simulink model "sampleModel1996"  (R2023a)
settings: Solver=VariableStepAuto  StartTime=0.0  StopTime=10.0  RelTol=1e-3
libraries: simulink x3, hdlsllib x2
settings Model: Creator=user1  LastModifiedBy=user1

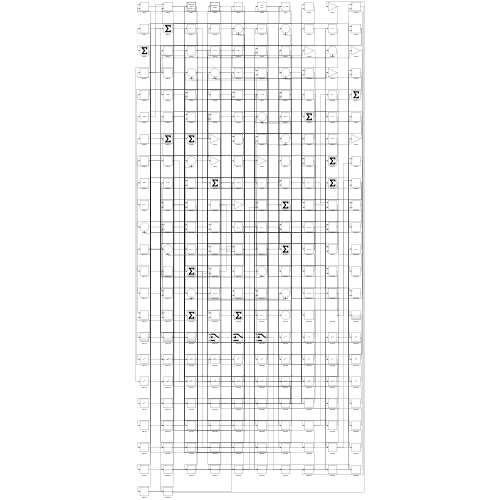
[thumbnail: Simulink's stored preview of the top-level diagram]
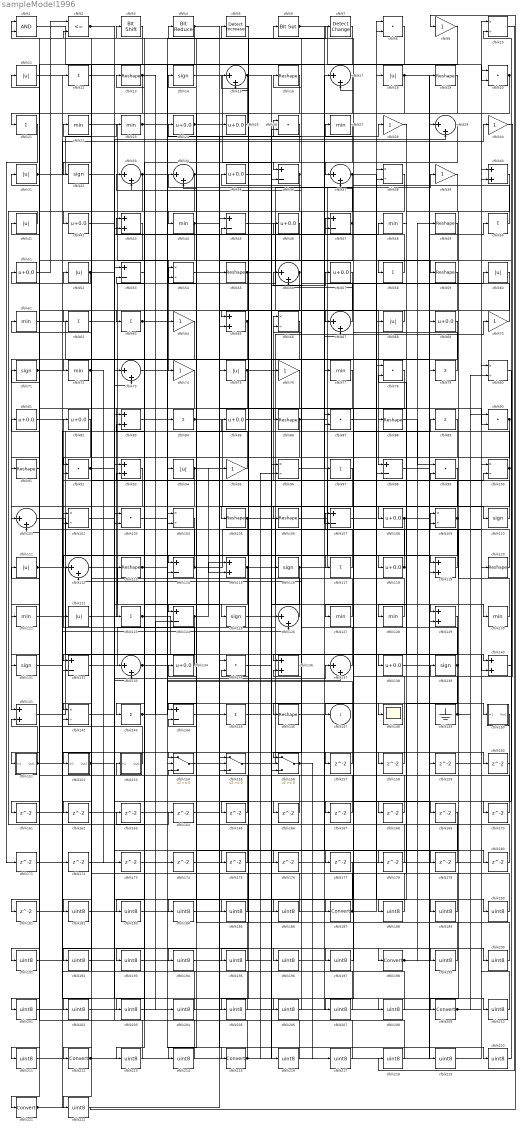
== system sampleModel1996 ==
  cfblk1 : Logic  AllPortsSameDT=off  OutDataTypeStr=boolean
  cfblk{10,38,54,66,80,96,100,102,104,109,142} (11 alike) : Product  Inputs=*/  RndMeth=Zero  SaturateOnIntegerOverflow=on
  cfblk{15,17,29,33..34,37,56,67,73,101,112,126,133,137} (14 alike) : Sum  Inputs=|++
  cfblk{8,20,26,78,87,90,92,99,103,135} (10 alike) : DotProduct  OutDataTypeStr=Inherit: Inherit via internal rule
  cfblk{13,16,19,49,55,59,86,88,91,105..106,113,120,146} (14 alike) : Reshape
  cfblk{36,45,47,53,98,107,114,124,132,144} (10 alike) : Sum  Inputs=+-
  cfblk{24..25,35,42,46,51,57,69,81..82,85,108,118,134,138} (15 alike) : Bias  Bias=0.0  SaturateOnIntegerOverflow=off
  cfblk{11,18,31,41,52,60,68,75,94,111,122} (11 alike) : Abs  SaturateOnIntegerOverflow=off
  cfblk{14,32,71,110,116,125,131,139} (8 alike) : Signum
  cfblk{40,43,65,83,93,115,119,129,136,140..141} (11 alike) : Sum
  cfblk{12,21,50,58,62..63,79,84,89,97,117,123,143,145} (14 alike) : Sum  Inputs=+
  cfblk{22..23,27,44,48,61,72,77,121,127..128,130} (12 alike) : MinMax
  cfblk148 : Scope
  cfblk149 : Ground
  cfblk150 : Subsystem
      settings: LibrarySourceBlock=|
      | hdlsllib/Ports &
      | Subsystems/Subsystem
  cfblk151 : Subsystem
      settings: LibrarySourceBlock=|
      | hdlsllib/Ports &
      | Subsystems/Subsystem
  cfblk152 : Subsystem
      settings: LibrarySourceBlock=|
      | hdlsllib/Ports &
      | Subsystems/Subsystem
  cfblk153 : Subsystem
      settings: LibrarySourceBlock=|
      | hdlsllib/Ports &
      | Subsystems/Subsystem
  cfblk154 : Switch  SaturateOnIntegerOverflow=off  InputSameDT=off
  cfblk155 : Switch  SaturateOnIntegerOverflow=off  InputSameDT=off
  cfblk156 : Switch  SaturateOnIntegerOverflow=off  InputSameDT=off
  cfblk{157..181} (25 alike) : Delay  SampleTime=1
  cfblk{182..186,188..197,199..208,210..211,213..214,216..220,222} (35 alike) : DataTypeConversion  OutDataTypeStr=uint8  SaturateOnIntegerOverflow=off  RndMeth=Floor
  cfblk{187,198,209,212,215,221} (6 alike) : DataTypeConversion  SaturateOnIntegerOverflow=off  RndMeth=Floor
  cfblk2 : RelationalOperator  Operator=<=  OutDataTypeStr=boolean  InputSameDT=off
  cfblk{9,28,30,39,64,70,74,76,95} (9 alike) : Gain
  cfblk3 : hdlsllib/Logic and Bit Operations/Bit Shift  mode=Shift Left Logical  N=0
  cfblk4 : hdlsllib/Logic and Bit Operations/Bit Reduce  mode=AND
  cfblk5 : simulink/Logic and Bit Operations/Detect Increase  vinit=0.0  OutDataTypeStr=boolean
      settings: LibrarySourceBlock=|
      | hdlsllib/Logic and Bit
      | Operations/Detect
      | Increase
  cfblk6 : simulink/Logic and Bit Operations/Bit Set  iBit=0
      settings: LibrarySourceBlock=|
      | hdlsllib/Logic and Bit
      | Operations/Bit Set
  cfblk7 : simulink/Logic and Bit Operations/Detect Change  vinit=0  OutDataTypeStr=boolean
      settings: LibrarySourceBlock=|
      | hdlsllib/Logic and Bit
      | Operations/Detect
      | Change
  cfblk147 : Outport  VectorParamsAs1DForOutWhenUnconnected=off
  wires:
  cfblk26/1 -> cfblk36/1
  cfblk60/1 -> cfblk74/1
  cfblk51/1 -> cfblk12/1
  cfblk84/1 -> cfblk110/1, cfblk107/2
  cfblk140/1 -> cfblk58/1
  cfblk110/1 -> cfblk66/1
  cfblk105/1 -> cfblk130/1, cfblk112/1, cfblk168/1
  cfblk123/1 -> cfblk156/3, cfblk204/1
  cfblk24/1 -> cfblk114/1, cfblk25/1
  cfblk115/1 -> cfblk70/1, cfblk213/1
  cfblk56/1 -> cfblk144/1, cfblk142/1
  cfblk23/1 -> cfblk148/1, cfblk199/1
  cfblk96/1 -> cfblk119/1
  cfblk134/1 -> cfblk82/1
  cfblk122/1 -> cfblk39/1
  cfblk74/1 -> cfblk123/1
  cfblk130/1 -> cfblk109/1
  cfblk52/1 -> cfblk51/1, cfblk46/1, cfblk169/1
  cfblk64/1 -> cfblk141/1
  cfblk70/1 -> cfblk35/1
  cfblk45/1 -> cfblk98/1
  cfblk88/1 -> cfblk99/1
  cfblk48/1 -> cfblk138/1
  cfblk59/1 -> cfblk86/1
  cfblk22/1 -> cfblk64/1
  cfblk29/1 -> cfblk37/1
  cfblk95/1 -> cfblk4/1
  cfblk132/1 -> cfblk18/1
  cfblk119/1 -> cfblk41/1
  cfblk151/1(Out1) -> cfblk141/2, cfblk100/2
  cfblk16/1 -> cfblk121/1
  cfblk141/1 -> cfblk36/2
  cfblk44/1 -> cfblk143/1, cfblk87/2
  cfblk120/1 -> cfblk14/1
  cfblk103/1 -> cfblk89/1
  cfblk126/1 -> cfblk61/1
  cfblk112/1 -> cfblk145/1
  cfblk111/1 -> cfblk140/1, cfblk154/1, cfblk126/2
  cfblk69/1 -> cfblk72/1
  cfblk38/1 -> cfblk106/1
  cfblk137/1 -> cfblk24/1
  cfblk49/1 -> cfblk88/1
  cfblk61/1 -> cfblk109/2
  cfblk155/1 -> cfblk68/1
  cfblk31/1 -> cfblk23/1, cfblk2/1, cfblk30/1
  cfblk58/1 -> cfblk3/1
  cfblk108/1 -> cfblk50/1, cfblk114/2
  cfblk9/1 -> cfblk221/1
  cfblk43/1 -> cfblk151/1(In1)
  cfblk79/1 -> cfblk34/1
  cfblk30/1 -> cfblk139/1
  cfblk72/1 -> cfblk173/1, cfblk222/1
  cfblk25/1 -> cfblk21/1
  cfblk150/1(Out1) -> cfblk153/1(In1)
  cfblk138/1 -> cfblk19/1
  cfblk144/1 -> cfblk45/1
  cfblk142/1 -> cfblk137/1
  cfblk154/1 -> cfblk26/1
  cfblk118/1 -> cfblk81/1, cfblk54/1
  cfblk153/1(Out1) -> cfblk111/1
  cfblk87/1 -> cfblk129/1
  cfblk4/1 -> cfblk59/1, cfblk154/2
  cfblk97/1 -> cfblk136/1
  cfblk94/1 -> cfblk115/2, cfblk180/1, cfblk181/1
  cfblk14/1 -> cfblk126/1
  cfblk149/1 -> cfblk1/1, cfblk80/2
  cfblk81/1 -> cfblk113/1
  cfblk113/1 -> cfblk43/1, cfblk99/2
  cfblk75/1 -> cfblk101/1, cfblk90/2, cfblk192/1
  cfblk6/1 -> cfblk20/2, cfblk67/2
  cfblk106/1 -> cfblk118/1
  cfblk63/1 -> cfblk28/1, cfblk7/1
  cfblk65/1 -> cfblk104/2, cfblk101/2
  cfblk117/1 -> cfblk71/1
  cfblk156/1 -> cfblk66/2, cfblk217/1
  cfblk116/1 -> cfblk60/1, cfblk156/2
  cfblk39/1 -> cfblk108/1
  cfblk86/1 -> cfblk29/1, cfblk152/1(In1)
  cfblk46/1 -> cfblk105/1
  cfblk3/1 -> cfblk32/1
  cfblk82/1 -> cfblk92/1
  cfblk28/1 -> cfblk128/1
  cfblk139/1 -> cfblk112/2, cfblk179/1, cfblk188/1
  cfblk90/1 -> cfblk147/1, cfblk142/2
  cfblk127/1 -> cfblk13/1
  cfblk109/1 -> cfblk22/1, cfblk156/1
  cfblk135/1 -> cfblk198/1
  cfblk143/1 -> cfblk94/1, cfblk124/2
  cfblk68/1 -> cfblk65/1
  cfblk136/1 -> cfblk56/1
  cfblk124/1 -> cfblk115/1, cfblk162/1
  cfblk27/1 -> cfblk63/1
  cfblk20/1 -> cfblk103/2, cfblk205/1
  cfblk47/1 -> cfblk15/1, cfblk132/1
  cfblk91/1 -> cfblk31/1
  cfblk101/1 -> cfblk119/2
  cfblk129/1 -> cfblk146/1
  cfblk13/1 -> cfblk92/2, cfblk84/1
  cfblk83/1 -> cfblk215/1
  cfblk66/1 -> cfblk125/1
  cfblk19/1 -> cfblk42/1
  cfblk152/1(Out1) -> cfblk29/2, cfblk196/1
  cfblk15/1 -> cfblk117/1, cfblk132/2
  cfblk2/1 -> cfblk176/1, cfblk177/1
  cfblk78/1 -> cfblk187/1
  cfblk35/1 -> cfblk116/1
  cfblk37/1 -> cfblk160/1, cfblk202/1
  cfblk50/1 -> cfblk27/1
  cfblk85/1 -> cfblk57/1
  cfblk11/1 -> cfblk155/2
  cfblk18/1 -> cfblk140/2, cfblk44/1
  cfblk55/1 -> cfblk91/1, cfblk129/2
  cfblk100/1 -> cfblk47/1, cfblk127/1
  cfblk121/1 -> cfblk85/1
  cfblk40/1 -> cfblk209/1
  cfblk133/1 -> cfblk48/1, cfblk137/2
  cfblk36/1 -> cfblk131/1, cfblk54/2
  cfblk114/1 -> cfblk52/1, cfblk80/1
  cfblk67/1 -> cfblk33/2
  cfblk62/1 -> cfblk124/1
  cfblk71/1 -> cfblk197/1, cfblk208/1
  cfblk92/1 -> cfblk133/1, cfblk2/2, cfblk133/2
  cfblk33/1 -> cfblk62/1, cfblk174/1, cfblk210/1
  cfblk34/1 -> cfblk67/1, cfblk150/1(In1), cfblk211/1
  cfblk1/1 -> cfblk97/1
  cfblk128/1 -> cfblk107/1
  cfblk93/1 -> cfblk212/1
  cfblk131/1 -> cfblk157/1
  cfblk157/1 -> cfblk104/1
  cfblk54/1 -> cfblk158/1
  cfblk158/1 -> cfblk56/2
  cfblk159/1 -> cfblk20/1
  cfblk99/1 -> cfblk161/1
  cfblk161/1 -> cfblk65/2
  cfblk163/1 -> cfblk33/1
  cfblk41/1 -> cfblk164/1
  cfblk57/1 -> cfblk165/1
  cfblk165/1 -> cfblk155/1
  cfblk12/1 -> cfblk166/1
  cfblk166/1 -> cfblk1/2
  cfblk145/1 -> cfblk167/1
  cfblk167/1 -> cfblk45/2
  cfblk168/1 -> cfblk103/1
  cfblk80/1 -> cfblk170/1
  cfblk170/1 -> cfblk144/2
  cfblk21/1 -> cfblk171/1
  cfblk171/1 -> cfblk43/2
  cfblk172/1 -> cfblk155/3
  cfblk173/1 -> cfblk100/1
  cfblk174/1 -> cfblk98/2
  cfblk32/1 -> cfblk175/1
  cfblk175/1 -> cfblk34/2
  cfblk176/1 -> cfblk38/2
  cfblk146/1 -> cfblk178/1
  cfblk178/1 -> cfblk15/2
  cfblk179/1 -> cfblk37/2
  cfblk180/1 -> cfblk136/2
  cfblk181/1 -> cfblk47/2
  cfblk8/1 -> cfblk182/1
  cfblk182/1 -> cfblk38/1
  cfblk104/1 -> cfblk183/1
  cfblk183/1 -> cfblk8/1
  cfblk177/1 -> cfblk184/1
  cfblk184/1 -> cfblk8/2
  cfblk5/1 -> cfblk185/1
  cfblk185/1 -> cfblk122/1
  cfblk42/1 -> cfblk186/1
  cfblk186/1 -> cfblk5/1
  cfblk187/1 -> cfblk96/1, cfblk154/3, cfblk87/1
  cfblk188/1 -> cfblk78/1
  cfblk107/1 -> cfblk189/1
  cfblk189/1 -> cfblk78/2
  cfblk73/1 -> cfblk190/1
  cfblk190/1 -> cfblk16/1
  cfblk7/1 -> cfblk191/1
  cfblk191/1 -> cfblk73/1
  cfblk192/1 -> cfblk73/2
  cfblk76/1 -> cfblk193/1
  cfblk193/1 -> cfblk95/1
  cfblk89/1 -> cfblk194/1
  cfblk194/1 -> cfblk76/1
  cfblk17/1 -> cfblk195/1
  cfblk195/1 -> cfblk134/1
  cfblk196/1 -> cfblk17/1
  cfblk197/1 -> cfblk17/2
  cfblk198/1 -> cfblk79/1, cfblk49/1
  cfblk199/1 -> cfblk135/1
  cfblk162/1 -> cfblk200/1
  cfblk200/1 -> cfblk135/2
  cfblk77/1 -> cfblk201/1
  cfblk201/1 -> cfblk55/1
  cfblk202/1 -> cfblk77/1
  cfblk53/1 -> cfblk203/1
  cfblk203/1 -> cfblk159/1
  cfblk204/1 -> cfblk53/1
  cfblk205/1 -> cfblk53/2
  cfblk102/1 -> cfblk206/1
  cfblk206/1 -> cfblk6/1
  cfblk160/1 -> cfblk207/1
  cfblk207/1 -> cfblk102/1
  cfblk208/1 -> cfblk102/2
  cfblk209/1 -> cfblk120/1, cfblk90/1
  cfblk210/1 -> cfblk40/1
  cfblk211/1 -> cfblk40/2
  cfblk212/1 -> cfblk26/2, cfblk69/1
  cfblk213/1 -> cfblk93/1
  cfblk169/1 -> cfblk214/1
  cfblk214/1 -> cfblk93/2
  cfblk215/1 -> cfblk163/1, cfblk96/2
  cfblk125/1 -> cfblk216/1
  cfblk216/1 -> cfblk83/1
  cfblk217/1 -> cfblk83/2
  cfblk10/1 -> cfblk218/1
  cfblk218/1 -> cfblk11/1
  cfblk98/1 -> cfblk219/1
  cfblk219/1 -> cfblk10/1
  cfblk164/1 -> cfblk220/1
  cfblk220/1 -> cfblk10/2
  cfblk221/1 -> cfblk172/1, cfblk75/1
  cfblk222/1 -> cfblk9/1

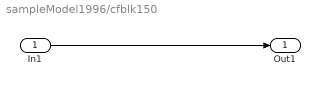
== system sampleModel1996/cfblk150 ==
  In1 : Inport
  Out1 : Outport
  wires:
  In1/1 -> Out1/1

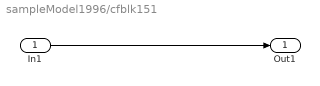
== system sampleModel1996/cfblk151 ==
  In1 : Inport
  Out1 : Outport
  wires:
  In1/1 -> Out1/1

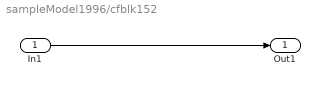
== system sampleModel1996/cfblk152 ==
  In1 : Inport
  Out1 : Outport
  wires:
  In1/1 -> Out1/1

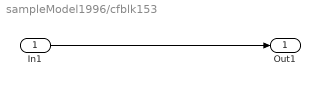
== system sampleModel1996/cfblk153 ==
  In1 : Inport
  Out1 : Outport
  wires:
  In1/1 -> Out1/1
